simulink model "read_FT60_2020a"  (R2020a)
settings: Solver=FixedStepAuto  StartTime=0.0  StopTime=60  RelTol=1e-3  EnableMultiTasking=on
values from neighbouring files (symbols this model uses):
  node = scgtnodestruct(node)    [initializeSCRAMNetGT.m]    (also in initializeSCRAMNetGT_com.m)
libraries: speedgoatlib_IO901_IO902 x2, slrtlib x1
settings Model: Creator=estructuras  LastModifiedBy=estructuras
settings SolverCC: ConcurrentTasks=on  PositivePriorityOrder=on  AutoInsertRateTranBlk=on
settings DataIOCC: SaveFormat=StructureWithTime
settings OptimizationCC: BlockReduction=off  OptimizeBlockIOStorage=off
settings DebuggingCC: TasksWithSamePriorityMsg=none  UnconnectedInputMsg=none  UnconnectedOutputMsg=none  UnconnectedLineMsg=none
settings HardwareCC: ProdBitPerPointer=32  ProdBitPerSizeT=32  ProdBitPerPtrDiffT=32  ProdLargestAtomicFloat=None  ProdWordSize=32  ProdLongLongMode=on  ProdHWDeviceType=Generic->32-bit x86 compatible
settings ModelReferenceCC: EnableRefExpFcnMdlSchedulingChecks=off
settings RTWCC: Description=Simulink Real-Time  SystemTargetFile=slrt.tlc  TemplateMakefile=slrt_default_tmf  BuildConfiguration=Faster Runs  CodeExecutionProfiling=on  RTWCompilerOptimization=on
settings SimulinkRealTimeCC: SupportVariableSizeSignals=on  RL32LogTETModifier=off  xPCConcurrentTasks=on

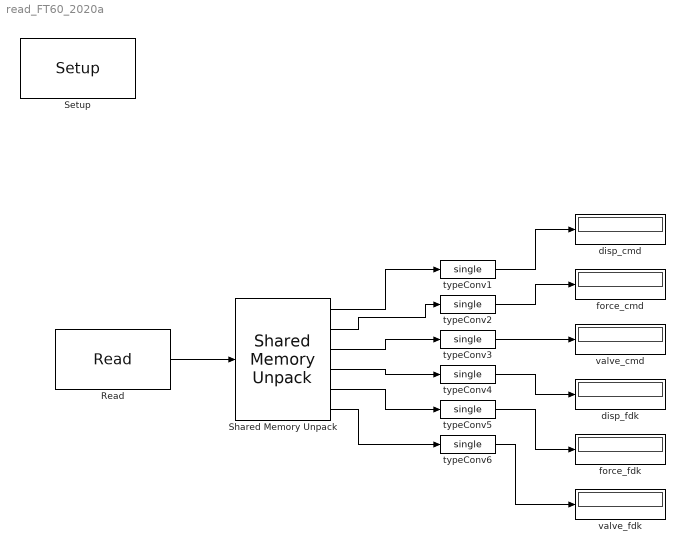
== system read_FT60_2020a ==
  "Read " : speedgoatlib_IO901_IO902/Read   id=1  partition=node.Partitions(8:13)  ts=0.001  pci=-1
      settings: SourceProductName=Simulink Real-Time: Speedgoat I/O Blockset
  "Setup " : speedgoatlib_IO901_IO902/Setup   id=1  node=node  pci=-1
      settings: SourceProductName=IO901 IO902
  "Shared Memory Unpack " : slrtlib/Shared Memory/Shared Memory Unpack   partition=node.Partitions(8:13)
      settings: SourceProductBaseCode=XP
  disp_cmd : Display
      settings: Decimation=3
  disp_fdk : Display
      settings: Decimation=3
  force_cmd : Display
      settings: Decimation=3
  force_fdk : Display
      settings: Decimation=3
  typeConv{1..6} (6 alike) : DataTypeConversion  OutDataTypeStr=single  SaturateOnIntegerOverflow=on  RndMeth=Zero
  valve_cmd : Display
      settings: Decimation=3
  valve_fdk : Display
      settings: Decimation=3
  wires:
  typeConv1/1 -> disp_cmd/1
  typeConv2/1 -> force_cmd/1
  typeConv3/1 -> valve_cmd/1
  typeConv4/1 -> disp_fdk/1
  typeConv5/1 -> force_fdk/1
  typeConv6/1 -> valve_fdk/1
  "Read "/1 -> "Shared Memory Unpack "/1
  "Shared Memory Unpack "/1 -> typeConv1/1
  "Shared Memory Unpack "/2 -> typeConv2/1
  "Shared Memory Unpack "/3 -> typeConv3/1
  "Shared Memory Unpack "/4 -> typeConv4/1
  "Shared Memory Unpack "/5 -> typeConv5/1
  "Shared Memory Unpack "/6 -> typeConv6/1
